simulink model "simulink_model"  (R2023b)
settings: Solver=VariableStepAuto  StartTime=0.0  StopTime=1.04  RelTol=1e-3
values from neighbouring files (symbols this model uses):
  k1 = -6    [parameters.m]
  k2 = -10    [parameters.m]
  k3 = 5    [parameters.m]
  k4 = 0.5    [parameters.m]
  k5 = -8    [parameters.m]
  kp_2 = -0.01    [parameters.m]
  t1 = 1.8    [parameters.m]
  t2 = 1    [parameters.m]
  t3 = 0.2    [parameters.m]
  t4 = 0.2    [parameters.m]
  t5 = 0.05    [parameters.m]
  td_2 = 4000    [parameters.m]
  ti_2 = 14000    [parameters.m]
libraries: simulink x3, slpidlib x2
settings Model: Creator=olavhegg  LastModifiedBy=olavhegg

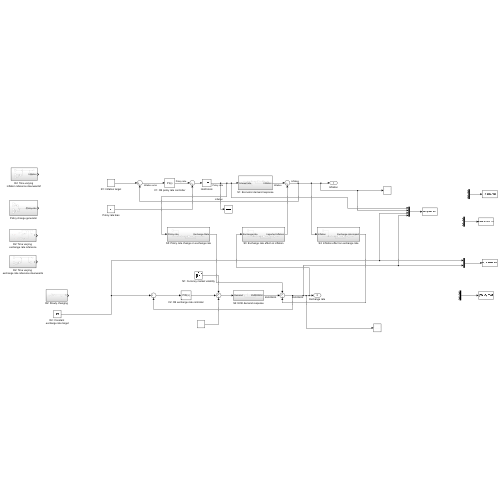
[thumbnail: Simulink's stored preview of the top-level diagram]
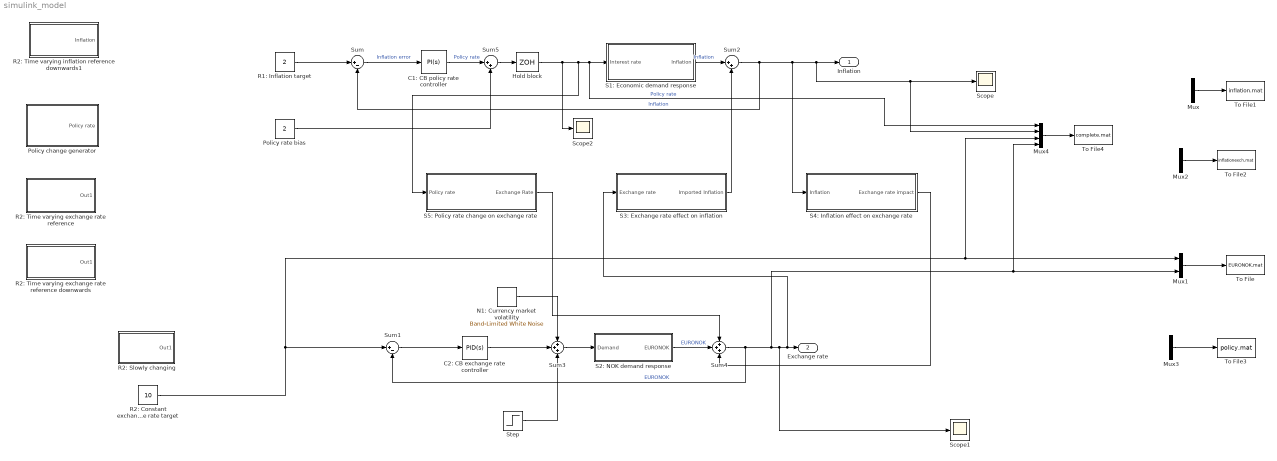
== system simulink_model ==
  C1: CB policy rate controller : slpidlib/PID Controller  Controller=PI  Form=Ideal  TimeDomain=Continuous-time  UseExternalTs=off  SampleTime=-1  IntegratorMethod=Forward Euler  FilterMethod=Forward Euler  ControllerParametersSource=internal  P=-2.2  I=3  UseKiTs=off  D=0  N=100  UseFilter=on  TunerSelectOption=Transfer Function Based (PID Tuner App)  InitialConditionSource=internal  InitialConditionForIntegrator=0  InitialConditionForFilter=0  DifferentiatorICPrevScaledInput=0  ExternalReset=none  TrackingMode=off  Kt=1  LimitOutput=off  SatLimitsSource=internal  UpperSaturationLimit=inf  LowerSaturationLimit=-inf  LinearizeAsGain=on  AntiWindupMode=none  Kb=1  LimitIntegrator=off  UpperIntegratorSaturationLimit=inf  LowerIntegratorSaturationLimit=-inf  POutMin=[]  POutMax=[]  IOutMin=[]  IOutMax=[]  DOutMin=[]  DOutMax=[]  NOutMin=[]  NOutMax=[]  SumOutMin=[]  SumOutMax=[]  SaturationOutMin=[]  SaturationOutMax=[]  PParamMin=[]  PParamMax=[]  IParamMin=[]  IParamMax=[]  DParamMin=[]  DParamMax=[]  NParamMin=[]  NParamMax=[]  KbParamMin=[]  KbParamMax=[]  KtParamMin=[]  KtParamMax=[]  KbOutMin=[]  KbOutMax=[]  KtOutMin=[]  KtOutMax=[]  IntegratorOutMin=[]  IntegratorOutMax=[]  FilterOutMin=[]  FilterOutMax=[]  SumI1OutMin=[]  SumI1OutMax=[]  SumI2OutMin=[]  SumI2OutMax=[]  SumI3OutMin=[]  SumI3OutMax=[]  SumI4OutMin=[]  SumI4OutMax=[]  SumDOutMin=[]  SumDOutMax=[]  DifferentiatorOutMin=[]  DifferentiatorOutMax=[]  FilterDiffOutCoefMin=[]  FilterDiffOutCoefMax=[]  ReciprocalOutMin=[]  ReciprocalOutMax=[]  SumDenOutMin=[]  SumDenOutMax=[]  SumNumOutMin=[]  SumNumOutMax=[]  DivideOutMin=[]  DivideOutMax=[]  UdiffTsProdOutMin=[]  UdiffTsProdOutMax=[]  NTsProdOutMin=[]  NTsProdOutMax=[]  UintegralTsProdOutMin=[]  UintegralTsProdOutMax=[]  UngainTsProdOutMin=[]  UngainTsProdOutMax=[]  ClampingZeroOutDataTypeStr=Inherit: Inherit via back propagation  ClampingZeroOutMin=[]  ClampingZeroOutMax=[]  FilterDenConstantOutDataTypeStr=Inherit: Inherit via back propagation  FilterDenConstantOutMin=[]  FilterDenConstantOutMax=[]  PCopyOutDataTypeStr=Inherit: Inherit via back propagation  PCopyOutMin=[]  PCopyOutMax=[]  NCopyOutDataTypeStr=Inherit: Inherit via back propagation  NCopyOutMin=[]  NCopyOutMax=[]  IntegratorContinuousStateAttributes=''  IntegratorStateMustResolveToSignalObject=off  IntegratorRTWStateStorageClass=Auto  FilterContinuousStateAttributes=''  FilterStateMustResolveToSignalObject=off  FilterRTWStateStorageClass=Auto  ParallelPVariant=Passthrough  IdealPVariant=InternalParameters  IVariant=InternalParameters  DVariant=Disabled  IntegratorVariant=Continuous  SatVariant=Disabled  AWVariant=Passthrough  PCopyVariant=Disabled  TRVariant=Disabled  FdbkBlocksVariant=Forward  IdealPFdbkVariant=Disabled  SatFdbkVariant=Disabled  DerivativeFilterVariant=Disabled  NVariant=Disabled  NCopyVariant=Disabled_SignalSpec  FilterICVariant=Disabled  IntegratorICVariant=InternalICs  ExternalResetVariant=Disabled  TRSumVariant=Passthrough  SumFdbkVariant=Disabled  SumVariant=Sum_PI  TsampFilterVariant=InternalTs  TsampNgainVariant=Passthrough  TsampIntegralVariant=Disabled_SignalSpec  ExternalSaturationOutDataTypeStr=Inherit: Same as second input
  C2: CB exchange rate controller : slpidlib/PID Controller  Controller=PID  Form=Ideal  TimeDomain=Continuous-time  UseExternalTs=off  SampleTime=-1  IntegratorMethod=Forward Euler  FilterMethod=Forward Euler  ControllerParametersSource=internal  P=kp_2  I=ti_2  UseKiTs=on  D=td_2  N=1  UseFilter=on  TunerSelectOption=Transfer Function Based (PID Tuner App)  InitialConditionSource=internal  InitialConditionForIntegrator=0  InitialConditionForFilter=0  DifferentiatorICPrevScaledInput=0  ExternalReset=none  TrackingMode=off  Kt=1  LimitOutput=off  SatLimitsSource=internal  UpperSaturationLimit=inf  LowerSaturationLimit=-inf  LinearizeAsGain=on  AntiWindupMode=none  Kb=1  LimitIntegrator=off  UpperIntegratorSaturationLimit=inf  LowerIntegratorSaturationLimit=-inf  POutMin=[]  POutMax=[]  IOutMin=[]  IOutMax=[]  DOutMin=[]  DOutMax=[]  NOutMin=[]  NOutMax=[]  SumOutMin=[]  SumOutMax=[]  SaturationOutMin=[]  SaturationOutMax=[]  PParamMin=[]  PParamMax=[]  IParamMin=[]  IParamMax=[]  DParamMin=[]  DParamMax=[]  NParamMin=[]  NParamMax=[]  KbParamMin=[]  KbParamMax=[]  KtParamMin=[]  KtParamMax=[]  KbOutMin=[]  KbOutMax=[]  KtOutMin=[]  KtOutMax=[]  IntegratorOutMin=[]  IntegratorOutMax=[]  FilterOutMin=[]  FilterOutMax=[]  SumI1OutMin=[]  SumI1OutMax=[]  SumI2OutMin=[]  SumI2OutMax=[]  SumI3OutMin=[]  SumI3OutMax=[]  SumI4OutMin=[]  SumI4OutMax=[]  SumDOutMin=[]  SumDOutMax=[]  DifferentiatorOutMin=[]  DifferentiatorOutMax=[]  FilterDiffOutCoefMin=[]  FilterDiffOutCoefMax=[]  ReciprocalOutMin=[]  ReciprocalOutMax=[]  SumDenOutMin=[]  SumDenOutMax=[]  SumNumOutMin=[]  SumNumOutMax=[]  DivideOutMin=[]  DivideOutMax=[]  UdiffTsProdOutMin=[]  UdiffTsProdOutMax=[]  NTsProdOutMin=[]  NTsProdOutMax=[]  UintegralTsProdOutMin=[]  UintegralTsProdOutMax=[]  UngainTsProdOutMin=[]  UngainTsProdOutMax=[]  ClampingZeroOutDataTypeStr=Inherit: Inherit via back propagation  ClampingZeroOutMin=[]  ClampingZeroOutMax=[]  FilterDenConstantOutDataTypeStr=Inherit: Inherit via back propagation  FilterDenConstantOutMin=[]  FilterDenConstantOutMax=[]  PCopyOutDataTypeStr=Inherit: Inherit via back propagation  PCopyOutMin=[]  PCopyOutMax=[]  NCopyOutDataTypeStr=Inherit: Inherit via back propagation  NCopyOutMin=[]  NCopyOutMax=[]  IntegratorContinuousStateAttributes=''  IntegratorStateMustResolveToSignalObject=off  IntegratorRTWStateStorageClass=Auto  FilterContinuousStateAttributes=''  FilterStateMustResolveToSignalObject=off  FilterRTWStateStorageClass=Auto  ParallelPVariant=Passthrough  IdealPVariant=InternalParameters  IVariant=InternalParameters  DVariant=InternalParameters  IntegratorVariant=Continuous  SatVariant=Disabled  AWVariant=Passthrough  PCopyVariant=Disabled  TRVariant=Disabled  FdbkBlocksVariant=Forward  IdealPFdbkVariant=Disabled  SatFdbkVariant=Disabled  DerivativeFilterVariant=ContFilter  NVariant=InternalParameters  NCopyVariant=Disabled  FilterICVariant=InternalICsFilter  IntegratorICVariant=InternalICs  ExternalResetVariant=Disabled  TRSumVariant=Passthrough  SumFdbkVariant=Disabled  SumVariant=Sum_PID  TsampFilterVariant=InternalTs  TsampNgainVariant=Passthrough  TsampIntegralVariant=Disabled_SignalSpec  ExternalSaturationOutDataTypeStr=Inherit: Same as second input
  Hold block : ZeroOrderHold  SampleTime=0.06
  Mux{,1..3} (4 alike) : Mux  Inputs=2
  Mux4 : Mux
  N1: Currency market volatility : simulink/Sources/Band-Limited White Noise  Cov=[0.002]  Ts=0.001  seed=[23341]
  Policy change generator : Subsystem
  Policy rate bias : Constant  Value=2
  R1: Inflation target : Constant  Value=2
  R2: Constant exchange rate target : Constant  Value=10
  R2: Slowly changing : Subsystem
  R2: Time varying exchange rate reference : Subsystem
  R2: Time varying exchange rate reference downwards : Subsystem
  R2: Time varying inflation reference downwards1 : Subsystem
  S1: Economic demand response : Subsystem
  S2: NOK demand response : Subsystem
  S3: Exchange rate effect on inflation : Subsystem
  S4: Inflation effect on exchange rate : Subsystem
  S5: Policy rate change on exchange rate : Subsystem
  Scope : Scope
  Scope1 : Scope
  Scope2 : Scope
  Step : Step  Time=0.4  After=-10  SampleTime=0
  Sum : Sum  Inputs=|+-
  Sum1 : Sum  Inputs=|+-
  Sum2 : Sum  Inputs=|++
  Sum3 : Sum  Inputs=+++
  Sum4 : Sum  Inputs=+++
  Sum5 : Sum  Inputs=|++
  To File : ToFile  Filename=EURONOK.mat  MatrixName=ERData
  To File1 : ToFile  Filename=inflation.mat  MatrixName=inflationData
  To File2 : ToFile  Filename=inflationexch.mat  MatrixName=inflationData
  To File3 : ToFile  Filename=policy.mat  MatrixName=policyData
  To File4 : ToFile  Filename=complete.mat  MatrixName=completeData
  Inflation : Outport
  Exchange rate : Outport  Port=2
  wires:
  R1: Inflation target/1 -> Sum/1
  Sum4/1 -> Mux4/4, Mux1/2, Scope1/1, S3: Exchange rate effect on inflation/1(Exchange rate), Exchange rate/1, Sum1/2  "EURONOK"
  C1: CB policy rate controller/1 -> Sum5/1  "Policy rate"
  Sum/1 -> C1: CB policy rate controller/1  "Inflation error"
  Sum3/1 -> S2: NOK demand response/1(Demand)
  C2: CB exchange rate controller/1 -> Sum3/2
  Sum2/1 -> Sum/2, Mux4/2, Scope/1, Inflation/1, S4: Inflation effect on exchange rate/1(Inflation)  "Inflation"
  N1: Currency market volatility/1 -> Sum3/1
  Sum1/1 -> C2: CB exchange rate controller/1
  Mux/1 -> To File1/1
  Mux1/1 -> To File/1
  Hold block/1 -> Scope2/1, Mux4/1, S1: Economic demand response/1(Interest rate), S5: Policy rate change on exchange rate/1(Policy rate)  "Policy rate"
  S1: Economic demand response/1(Inflation) -> Sum2/1  "Inflation"
  S3: Exchange rate effect on inflation/1(Imported Inflation) -> Sum2/2
  S4: Inflation effect on exchange rate/1(Exchange rate impact) -> Sum4/3
  Mux2/1 -> To File2/1
  S5: Policy rate change on exchange rate/1(Exchange Rate) -> Sum4/1
  Mux3/1 -> To File3/1
  S2: NOK demand response/1(EURONOK) -> Sum4/2  "EURONOK"
  R2: Constant exchange rate target/1 -> Mux4/3, Mux1/1, Sum1/1
  Sum5/1 -> Hold block/1
  Policy rate bias/1 -> Sum5/2
  Mux4/1 -> To File4/1
  Step/1 -> Sum3/3

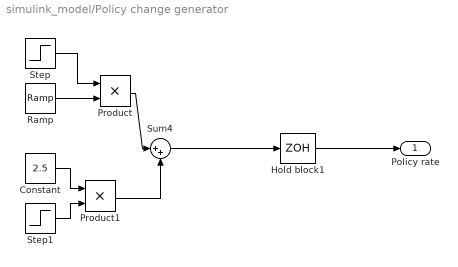
== system simulink_model/Policy change generator ==
  Constant : Constant  Value=2.5
  Hold block1 : ZeroOrderHold  SampleTime=0.06
  Product : Product
  Product1 : Product
  Ramp : simulink/Sources/Ramp  slope=2  start=0.4  InitialOutput=2
  Step : Step  Time=0.65  Before=1  After=0  SampleTime=0
  Step1 : Step  Time=0.65  SampleTime=0
  Sum4 : Sum  Inputs=|++
  Policy rate : Outport
  wires:
  Constant/1 -> Product1/1
  Step/1 -> Product/1
  Sum4/1 -> Hold block1/1
  Product/1 -> Sum4/1
  Ramp/1 -> Product/2
  Hold block1/1 -> Policy rate/1
  Product1/1 -> Sum4/2
  Step1/1 -> Product1/2

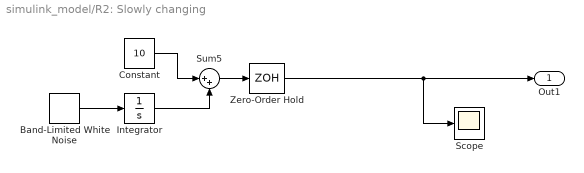
== system simulink_model/R2: Slowly changing ==
  Band-Limited White Noise : simulink/Sources/Band-Limited White Noise  Cov=[0.1]  Ts=0.2  seed=[233421]
  Constant : Constant  Value=10
  Integrator : Integrator
  Scope : Scope
  Sum5 : Sum  Inputs=|++
  Zero-Order Hold : ZeroOrderHold  SampleTime=0.01
  Out1 : Outport
  wires:
  Integrator/1 -> Sum5/2
  Band-Limited White Noise/1 -> Integrator/1
  Sum5/1 -> Zero-Order Hold/1
  Constant/1 -> Sum5/1
  Zero-Order Hold/1 -> Scope/1, Out1/1

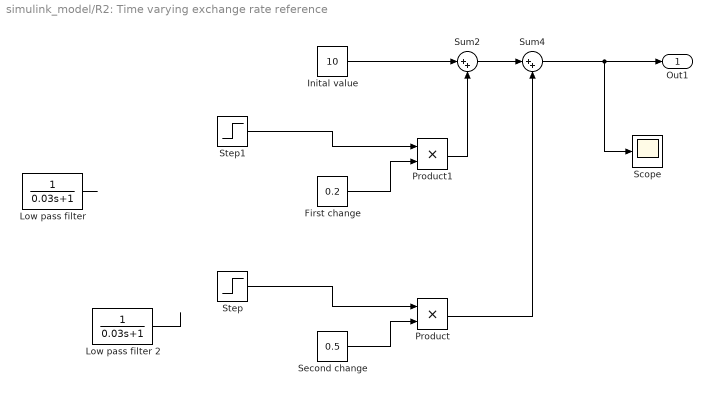
== system simulink_model/R2: Time varying exchange rate reference ==
  First change : Constant  Value=0.2
  Inital value : Constant  Value=10
  Low pass filter : TransferFcn  Denominator=[0.03 1]
  Low pass filter 2 : TransferFcn  Denominator=[0.03 1]
  Product : Product
  Product1 : Product
  Scope : Scope
  Second change : Constant  Value=0.5
  Step : Step  Time=0.70  SampleTime=0
  Step1 : Step  Time=0.40  SampleTime=0
  Sum2 : Sum  Inputs=|++
  Sum4 : Sum  Inputs=|++
  Out1 : Outport
  wires:
  Inital value/1 -> Sum2/1
  Product/1 -> Sum4/2
  Second change/1 -> Product/2
  Step/1 -> Product/1
  Sum2/1 -> Sum4/1
  Product1/1 -> Sum2/2
  First change/1 -> Product1/2
  Step1/1 -> Product1/1
  Sum4/1 -> Scope/1, Out1/1
  Low pass filter/1 -> ?
  Low pass filter 2/1 -> ?

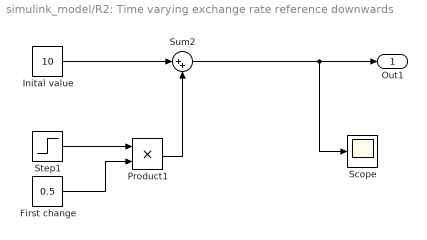
== system simulink_model/R2: Time varying exchange rate reference downwards ==
  First change : Constant  Value=0.5
  Inital value : Constant  Value=10
  Product1 : Product
  Scope : Scope
  Step1 : Step  Time=0.40  SampleTime=0
  Sum2 : Sum  Inputs=|++
  Out1 : Outport
  wires:
  Inital value/1 -> Sum2/1
  Product1/1 -> Sum2/2
  First change/1 -> Product1/2
  Step1/1 -> Product1/1
  Sum2/1 -> Scope/1, Out1/1

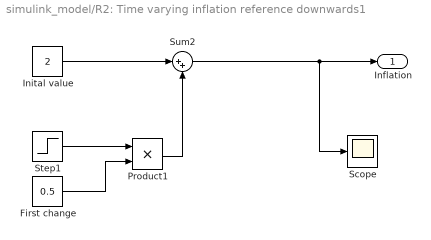
== system simulink_model/R2: Time varying inflation reference downwards1 ==
  First change : Constant  Value=0.5
  Inital value : Constant  Value=2
  Product1 : Product
  Scope : Scope
  Step1 : Step  Time=0.40  SampleTime=0
  Sum2 : Sum  Inputs=|++
  Inflation : Outport
  wires:
  Inital value/1 -> Sum2/1
  Product1/1 -> Sum2/2
  First change/1 -> Product1/2
  Step1/1 -> Product1/1
  Sum2/1 -> Scope/1, Inflation/1

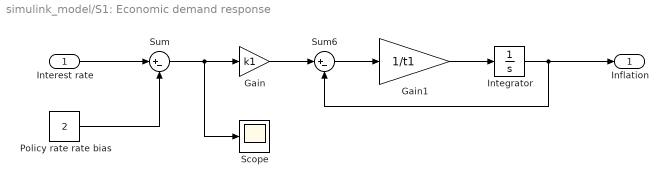
== system simulink_model/S1: Economic demand response ==
  Interest rate : Inport
  Gain : Gain  Gain=k1
  Gain1 : Gain  Gain=1/t1
  Integrator : Integrator  InitialCondition=2
  Policy rate rate bias : Constant  Value=2
  Scope : Scope
  Sum : Sum  Inputs=|+-
  Sum6 : Sum  Inputs=|+-
  Inflation : Outport
  wires:
  Integrator/1 -> Inflation/1, Sum6/2
  Interest rate/1 -> Sum/1
  Gain/1 -> Sum6/1
  Gain1/1 -> Integrator/1
  Sum6/1 -> Gain1/1
  Policy rate rate bias/1 -> Sum/2
  Sum/1 -> Scope/1, Gain/1

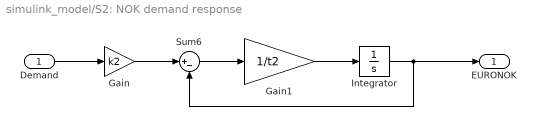
== system simulink_model/S2: NOK demand response ==
  Demand : Inport
  Gain : Gain  Gain=k2
  Gain1 : Gain  Gain=1/t2
  Integrator : Integrator  InitialCondition=10
  Sum6 : Sum  Inputs=|+-
  EURONOK : Outport
  wires:
  Integrator/1 -> EURONOK/1, Sum6/2
  Demand/1 -> Gain/1
  Gain/1 -> Sum6/1
  Gain1/1 -> Integrator/1
  Sum6/1 -> Gain1/1

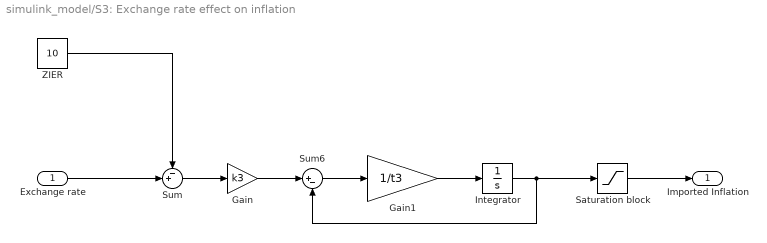
== system simulink_model/S3: Exchange rate effect on inflation ==
  Exchange rate : Inport
  Gain : Gain  Gain=k3
  Gain1 : Gain  Gain=1/t3
  Integrator : Integrator
  Saturation block : Saturate
  Sum : Sum  Inputs=-+|
  Sum6 : Sum  Inputs=|+-
  ZIER : Constant  Value=10
  Imported Inflation : Outport
  wires:
  Integrator/1 -> Saturation block/1, Sum6/2
  Gain/1 -> Sum6/1
  Gain1/1 -> Integrator/1
  Sum6/1 -> Gain1/1
  Exchange rate/1 -> Sum/2
  ZIER/1 -> Sum/1
  Sum/1 -> Gain/1
  Saturation block/1 -> Imported Inflation/1

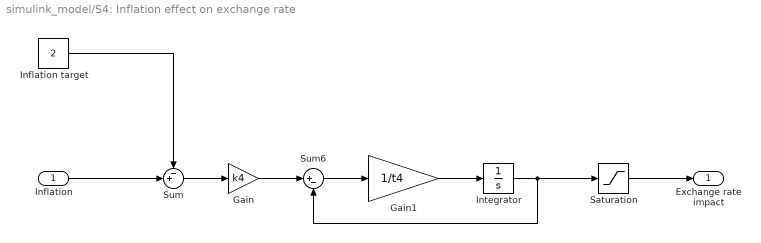
== system simulink_model/S4: Inflation effect on exchange rate ==
  Inflation : Inport
  Gain : Gain  Gain=k4
  Gain1 : Gain  Gain=1/t4
  Inflation target : Constant  Value=2
  Integrator : Integrator
  Saturation : Saturate
  Sum : Sum  Inputs=-+|
  Sum6 : Sum  Inputs=|+-
  Exchange rate impact : Outport
  wires:
  Gain/1 -> Sum6/1
  Gain1/1 -> Integrator/1
  Sum6/1 -> Gain1/1
  Inflation/1 -> Sum/2
  Inflation target/1 -> Sum/1
  Sum/1 -> Gain/1
  Integrator/1 -> Sum6/2, Saturation/1
  Saturation/1 -> Exchange rate impact/1

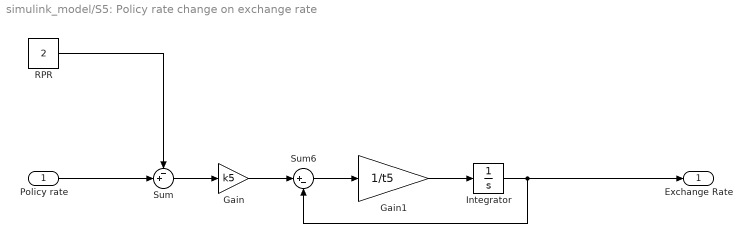
== system simulink_model/S5: Policy rate change on exchange rate ==
  Policy rate : Inport
  Gain : Gain  Gain=k5
  Gain1 : Gain  Gain=1/t5
  Integrator : Integrator
  RPR : Constant  Value=2
  Sum : Sum  Inputs=-+|
  Sum6 : Sum  Inputs=|+-
  Exchange Rate : Outport
  wires:
  Gain/1 -> Sum6/1
  Gain1/1 -> Integrator/1
  Sum6/1 -> Gain1/1
  Policy rate/1 -> Sum/2
  RPR/1 -> Sum/1
  Sum/1 -> Gain/1
  Integrator/1 -> Exchange Rate/1, Sum6/2
